simulink model "SRM"  (R2023a)
settings: Solver=VariableStepAuto  StartTime=0.0  StopTime=0.03  RelTol=1e-3
undefined symbols (not defined in the file): DiscIntNeverNeededParam, Ts
libraries: spsDiodeLib x6, spsIGBTLib x6, spsDCVoltageSourceLib x1, spsSwitchedReluctanceMotorLib x1, sps_lib x1
settings Model: Creator=Hp  LastModifiedBy=Hp

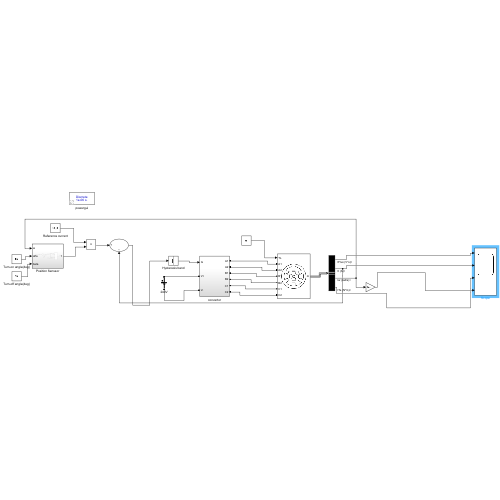
[thumbnail: Simulink's stored preview of the top-level diagram]
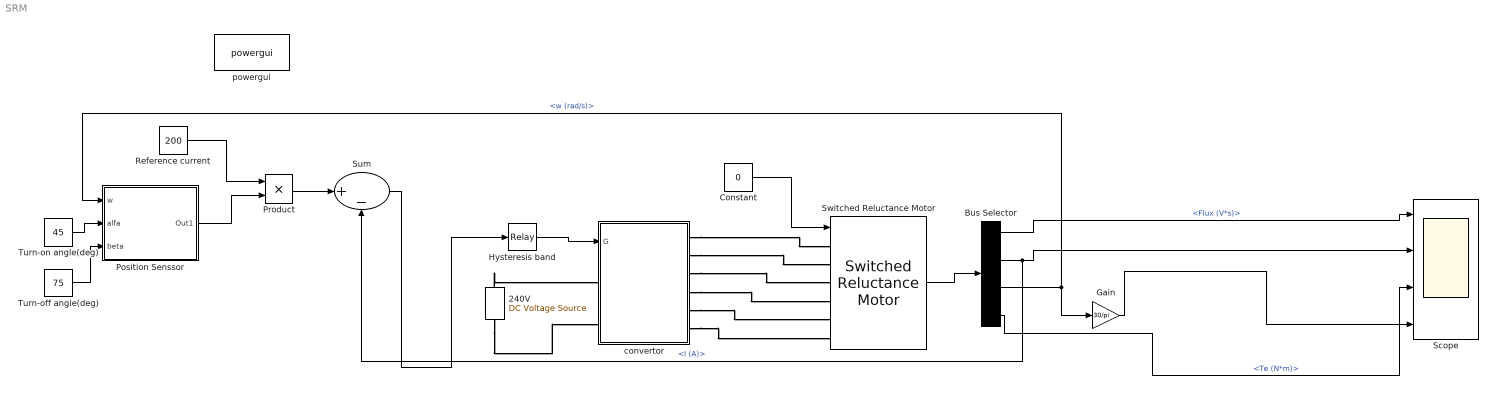
== system SRM ==
  240V : spsDCVoltageSourceLib/DC Voltage Source  Amplitude=240  Measurements=Voltage
  Bus Selector : BusSelector  OutputSignals=Flux (V*s),I (A),w (rad/s),Te (N*m)
  Constant : Constant  Value=0
  Gain : Gain  Gain=30/pi
  Hysteresis band : Relay  OnSwitchValue=10  OffSwitchValue=-10  InputProcessing=Columns as channels (frame based)  ZeroCross=off
  Position Senssor : Subsystem
  Product : Product
  Reference current : Constant  Value=200
  Scope : Scope  NumInputPorts=4
  Sum : Sum  Inputs=|+-
  Switched Reluctance Motor : spsSwitchedReluctanceMotorLib/Switched Reluctance Motor  MachineType="6/4  (60 kw preset model)"  StatorResistance=0.05  Inertia=0.05  Friction=0.2  InitialSpeed=[0 0]  TsPowergui=0  TsBlock=Ts  MachineModel=Specific model  Lq=0.67e-3  Ld=23.6e-3  Lsat=0.15e-3  MaximumCurrent=450  MaximumFluxLinkage=0.486  Source=Dialog  MagnetisationCharacteristic='srm64_60kw.mat'  RotorAngleVector=[0 10 20 30 40 45]  StatorCurrentVector=[0:25:450]  PlotCurves=off
      settings: LibrarySourceBlock=|
      | sps_lib/Electrical Machines/Switched Reluctance
      | Motor
  Turn-off angle(deg) : Constant  Value=75
  Turn-on angle(deg) : Constant  Value=45
  convertor : Subsystem
  powergui : sps_lib/powergui  Priority=1  SimulationMode=Discrete  SampleTime=1e-06  frequency=60  Iterations=50  frequencyindice=0  Pbase=100e6  ErrMax=1e-4  UnitsV=kV  UnitsW=MW  buscounter=0  FunctionMessages=off  echomessages=off  EnableUseOfTLC=off  CurrentSourceSwitches=off  DisableSnubberDevices=off  DisableRonSwitches=off  DisableVfSwitches=off  DisplayEquations=off  AutomaticDiscreteSolvers=off  SolverType=Tustin/Backward Euler (TBE)  Interpol=off  ExternalGateDelay=off  methode=off  Ts=100  x0status=blocks  SPID=on  SwTol=0  HookPort=off  NonlinearTolerance=1e-4  nMaxIteration=100  ContinueOnMaxIteration=off  RestoreLinks=warning  ResistiveCurrentMeasurement=off  Frange=[0:2:500]  Ylog=off  Xlog=on  ShowGrid=off  save=off  variable=ZData  structure=0  ZoomFFT=off  StartTime=0.0  cycles=1  DisplayStyle=1  fundamental=60  FreqAxis=off  MaxFrequency=1000  frequencyindicesteady=1  RmsSteady=1  display=off
  wires:
  Position Senssor/1(Out1) -> Product/2
  Product/1 -> Sum/1
  Turn-off angle(deg)/1 -> Position Senssor/3(beta)
  Sum/1 -> Hysteresis band/1
  Turn-on angle(deg)/1 -> Position Senssor/2(alfa)
  Constant/1 -> Switched Reluctance Motor/1
  Switched Reluctance Motor/1 -> Bus Selector/1
  Hysteresis band/1 -> convertor/1(G)
  Reference current/1 -> Product/1
  Bus Selector/3 -> Gain/1, Position Senssor/1(w)  "<w (rad/s)>"
  Bus Selector/2 -> Scope/2, Sum/2  "<I (A)>"
  Bus Selector/1 -> Scope/1  "<Flux (V*s)>"
  Bus Selector/4 -> Scope/3  "<Te (N*m)>"
  Gain/1 -> Scope/4
  connections:
  240V/LConn1 -- convertor/LConn2
  convertor/RConn4 -- Switched Reluctance Motor/LConn4
  convertor/RConn1 -- Switched Reluctance Motor/LConn1
  convertor/RConn3 -- Switched Reluctance Motor/LConn3
  240V/RConn1 -- convertor/LConn1
  convertor/RConn6 -- Switched Reluctance Motor/LConn6
  convertor/RConn5 -- Switched Reluctance Motor/LConn5
  convertor/RConn2 -- Switched Reluctance Motor/LConn2

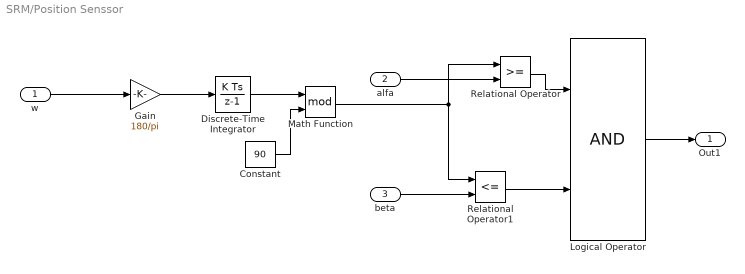
== system SRM/Position Senssor ==
  w : Inport
  alfa : Inport  Port=2
  beta : Inport  Port=3
  Constant : Constant  Value=90
  Discrete-Time Integrator : DiscreteIntegrator  InitialCondition=[0 -30 -60]  SampleTime=Ts  ICPrevOutput=DiscIntNeverNeededParam  ICPrevScaledInput=DiscIntNeverNeededParam
  Gain : Gain  Gain=180/pi
  Logical Operator : Logic  AllPortsSameDT=off  OutDataTypeStr=boolean
  Math Function : Math  Operator=mod
  Relational Operator : RelationalOperator  OutDataTypeStr=boolean  RndMeth=Simplest  InputSameDT=off
  Relational Operator1 : RelationalOperator  Operator=<=  OutDataTypeStr=boolean  RndMeth=Simplest  InputSameDT=off
  Out1 : Outport
  wires:
  w/1 -> Gain/1
  Gain/1 -> Discrete-Time Integrator/1
  Discrete-Time Integrator/1 -> Math Function/1
  Constant/1 -> Math Function/2
  Math Function/1 -> Relational Operator/1, Relational Operator1/1
  alfa/1 -> Relational Operator/2
  beta/1 -> Relational Operator1/2
  Relational Operator/1 -> Logical Operator/1
  Relational Operator1/1 -> Logical Operator/2
  Logical Operator/1 -> Out1/1

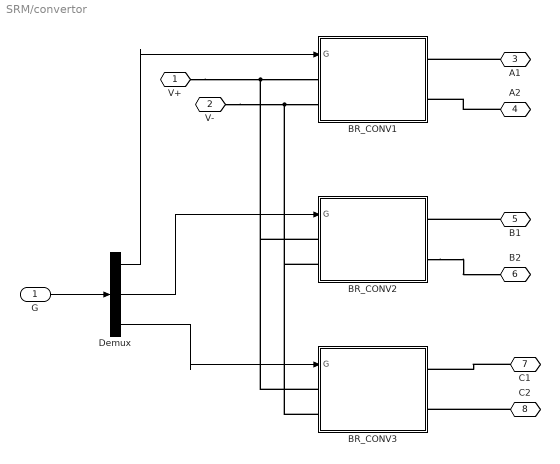
== system SRM/convertor ==
  G : Inport
  BR_CONV1 : Subsystem
  BR_CONV2 : Subsystem
  BR_CONV3 : Subsystem
  Demux : Demux  Outputs=3
  V+ : PMIOPort  Side=Left
  V- : PMIOPort  Port=2  Side=Left
  A1 : PMIOPort  Port=3  Side=Right
  A2 : PMIOPort  Port=4  Side=Right
  B1 : PMIOPort  Port=5  Side=Right
  B2 : PMIOPort  Port=6  Side=Right
  C1 : PMIOPort  Port=7  Side=Right
  C2 : PMIOPort  Port=8  Side=Right
  wires:
  G/1 -> Demux/1
  Demux/1 -> BR_CONV1/1(G)
  Demux/2 -> BR_CONV2/1(G)
  Demux/3 -> BR_CONV3/1(G)
  connections:
  V-/RConn1 -- BR_CONV3/LConn2 -- BR_CONV2/LConn2 -- BR_CONV1/LConn2
  V+/RConn1 -- BR_CONV3/LConn1 -- BR_CONV2/LConn1 -- BR_CONV1/LConn1
  A1/RConn1 -- BR_CONV1/RConn1
  A2/RConn1 -- BR_CONV1/RConn2
  BR_CONV2/RConn2 -- B2/RConn1
  B1/RConn1 -- BR_CONV2/RConn1
  C2/RConn1 -- BR_CONV3/RConn2
  C1/RConn1 -- BR_CONV3/RConn1

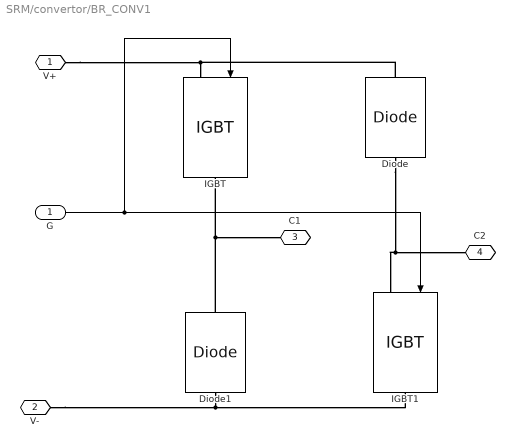
== system SRM/convertor/BR_CONV1 ==
  G : Inport
  Diode : spsDiodeLib/Diode  Ron=1E-3  Lon=0  Vf=0.8  IC=0  UseSnubber=0  Rs=1000  Cs=Inf  Measurements=off
  Diode1 : spsDiodeLib/Diode  Ron=1E-3  Lon=0  Vf=0.8  IC=0  UseSnubber=0  Rs=1000  Cs=Inf  Measurements=off
  IGBT : spsIGBTLib/IGBT  Ron=1E-3  Lon=0  Vf=1  Tf=1e-6  Tt=2e-6  IC=0  Rs=200  Cs=0.1E-06  Measurements=off
  IGBT1 : spsIGBTLib/IGBT  Ron=1E-3  Lon=0  Vf=1  Tf=1e-6  Tt=2e-6  IC=0  Rs=200  Cs=0.1E-06  Measurements=off
  V+ : PMIOPort  Side=Left
  V- : PMIOPort  Port=2  Side=Left
  C1 : PMIOPort  Port=3  Side=Right
  C2 : PMIOPort  Port=4  Side=Right
  wires:
  G/1 -> IGBT/1, IGBT1/1
  connections:
  Diode/RConn1 -- V+/RConn1 -- IGBT/LConn1
  Diode/LConn1 -- C2/RConn1 -- IGBT1/LConn1
  Diode1/LConn1 -- V-/RConn1 -- IGBT1/RConn1
  Diode1/RConn1 -- C1/RConn1 -- IGBT/RConn1

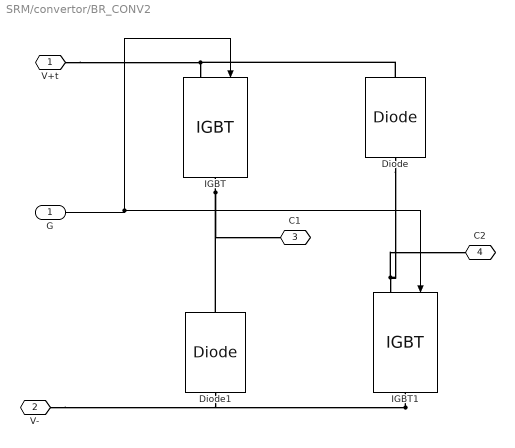
== system SRM/convertor/BR_CONV2 ==
  G : Inport
  Diode : spsDiodeLib/Diode  Ron=1E-3  Lon=0  Vf=0.8  IC=0  UseSnubber=0  Rs=1000  Cs=Inf  Measurements=off
  Diode1 : spsDiodeLib/Diode  Ron=1E-3  Lon=0  Vf=0.8  IC=0  UseSnubber=0  Rs=1000  Cs=Inf  Measurements=off
  IGBT : spsIGBTLib/IGBT  Ron=1E-3  Lon=0  Vf=1  Tf=1e-6  Tt=2e-6  IC=0  Rs=200  Cs=0.1E-06  Measurements=off
  IGBT1 : spsIGBTLib/IGBT  Ron=1E-3  Lon=0  Vf=1  Tf=1e-6  Tt=2e-6  IC=0  Rs=200  Cs=0.1E-06  Measurements=off
  V+t : PMIOPort  Side=Left
  V- : PMIOPort  Port=2  Side=Left
  C1 : PMIOPort  Port=3  Side=Right
  C2 : PMIOPort  Port=4  Side=Right
  wires:
  G/1 -> IGBT1/1, IGBT/1
  connections:
  IGBT/LConn1 -- Diode/RConn1 -- V+t/RConn1
  IGBT1/LConn1 -- Diode/LConn1 -- C2/RConn1
  IGBT1/RConn1 -- Diode1/LConn1 -- V-/RConn1
  IGBT/RConn1 -- Diode1/RConn1 -- C1/RConn1

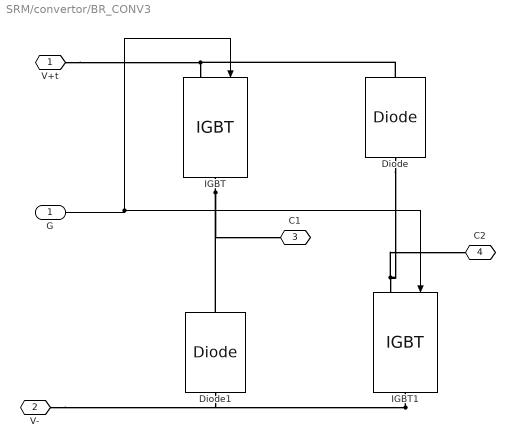
== system SRM/convertor/BR_CONV3 ==
  G : Inport
  Diode : spsDiodeLib/Diode  Ron=1E-3  Lon=0  Vf=0.8  IC=0  UseSnubber=0  Rs=1000  Cs=Inf  Measurements=off
  Diode1 : spsDiodeLib/Diode  Ron=1E-3  Lon=0  Vf=0.8  IC=0  UseSnubber=0  Rs=1000  Cs=Inf  Measurements=off
  IGBT : spsIGBTLib/IGBT  Ron=1E-3  Lon=0  Vf=1  Tf=1e-6  Tt=2e-6  IC=0  Rs=200  Cs=0.1E-06  Measurements=off
  IGBT1 : spsIGBTLib/IGBT  Ron=1E-3  Lon=0  Vf=1  Tf=1e-6  Tt=2e-6  IC=0  Rs=200  Cs=0.1E-06  Measurements=off
  V+t : PMIOPort  Side=Left
  V- : PMIOPort  Port=2  Side=Left
  C1 : PMIOPort  Port=3  Side=Right
  C2 : PMIOPort  Port=4  Side=Right
  wires:
  G/1 -> IGBT1/1, IGBT/1
  connections:
  IGBT/LConn1 -- Diode/RConn1 -- V+t/RConn1
  IGBT1/LConn1 -- Diode/LConn1 -- C2/RConn1
  IGBT1/RConn1 -- Diode1/LConn1 -- V-/RConn1
  IGBT/RConn1 -- Diode1/RConn1 -- C1/RConn1
